simulink model "BLDC_closed_P"  (Simulink 7.1)
settings: Solver=ode45  StartTime=0.0  StopTime=10  RelTol=1e-3
settings Model: Creator=Tang  LastModifiedBy=Tang

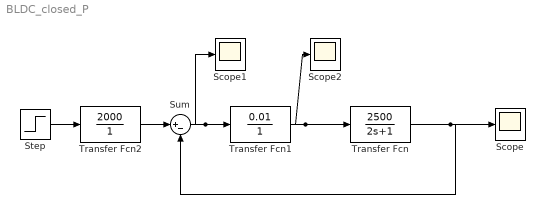
== system BLDC_closed_P ==
  Scope : Scope
  Scope1 : Scope
  Scope2 : Scope
      settings: SaveName=ScopeData2
  Step : Step  Time=0  SampleTime=0
  Sum : Sum  Inputs=|+-  OutDataType=sfix(16)  OutScaling=2^0
  Transfer Fcn : TransferFcn  Numerator=[2500]  Denominator=[2 1]
  Transfer Fcn1 : TransferFcn  Numerator=[0.01]  Denominator=[ 0 1]
  Transfer Fcn2 : TransferFcn  Numerator=[2000]  Denominator=[0 1]
  wires:
  Transfer Fcn/1 -> Scope/1, Sum/2
  Sum/1 -> Transfer Fcn1/1, Scope1/1
  Transfer Fcn1/1 -> Transfer Fcn/1, Scope2/1
  Transfer Fcn2/1 -> Sum/1
  Step/1 -> Transfer Fcn2/1
